simulink model "Controls_Finalproject_1f_linear"  (R2015a)
settings: Solver=ode45  StartTime=0.0  StopTime=1000.0  RelTol=1e-3
values from neighbouring files (symbols this model uses):
  A = [ 0 1 0 0 0 0; 0 0 -(m1*g)/M 0 -m2*g/M 0 ; 0 0 0 1 0 0 ; 0 0 -(M+m1)*g/(M*l1) 0 -m2*g/(M*l1) 0 ; 0 0 0 0 0 1; 0 0 -m1*g/(M*l2) 0 -(M+m2)*g/(M*l2) 0]    [linear_1f.m]    (also in nonlinear_1g.m = [ 0 1 0 0 0 0; 0 0 -(m1*g)/M 0 -m2*g/M 0; 0 0 0 1 0 0; 0 0 -)
  AKL = AKL1    [linear_1f.m]    (also in nonlinear_1g.m)
  B = [0; 1/M; 0; 1/(M*l1); 0; 1/(M*l2)]    [linear_1f.m]    (also in nonlinear_1g.m)
  BL = BL1    [linear_1f.m]    (also in nonlinear_1g.m)
  C = C1    [linear_1f.m]    (also in nonlinear_1g.m)
  CO = eye(6)    [linear_1f.m]    (also in nonlinear_1g.m)
  D = D1    [linear_1f.m]    (also in nonlinear_1g.m)
  DO = DO1    [linear_1f.m]    (also in nonlinear_1g.m)
  X0 = X01    [linear_1f.m]
undefined symbols (not defined in the file or in its folder): K
settings Model: Creator=Aditya Earanky  LastModifiedBy=Vishakha

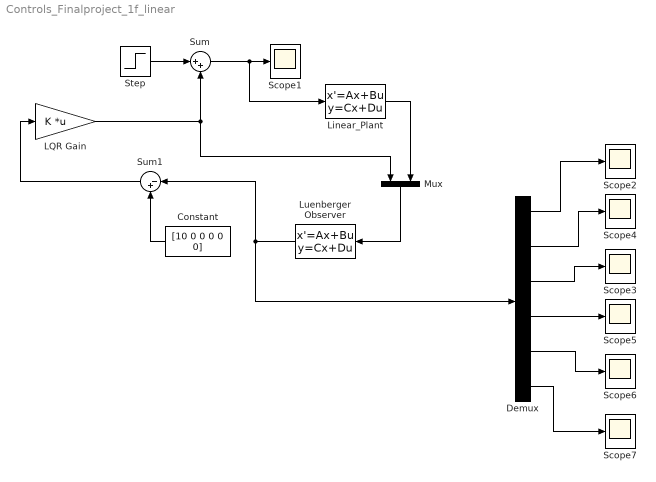
== system Controls_Finalproject_1f_linear ==
  Constant : Constant  Value=[10 0 0 0 0 0]
  Demux : Demux  Outputs=6
  LQR Gain : Gain  Gain=K  Multiplication=Matrix(K*u)
  Linear_Plant : StateSpace  A=A  B=B  C=C  D=D  X0=X0
  Luenberger Observer : StateSpace  A=AKL  B=BL  C=CO  D=DO  X0=0
  Mux : Mux  Inputs=2
  Scope{1..7} (7 alike) : Scope
      Scope1 settings: TimeRange=1000  YMin=0  YMax=0.07
      Scope2 settings: TimeRange=1000  YMin=0  YMax=0.07  SaveName=ScopeData2
      Scope3 settings: TimeRange=1000  YMin=0  YMax=0.07  SaveName=ScopeData3
      Scope4 settings: TimeRange=1000  YMin=0  YMax=0.07  SaveName=ScopeData4
      Scope5 settings: TimeRange=1000  YMin=0  YMax=0.07  SaveName=ScopeData5
      Scope6 settings: TimeRange=1000  YMin=0  YMax=0.07  SaveName=ScopeData6
      Scope7 settings: TimeRange=1000  YMin=0  YMax=0.07  SaveName=ScopeData7
  Step : Step  SampleTime=0
  Sum : Sum  Inputs=|++
  Sum1 : Sum  Inputs=|-+
  wires:
  Linear_Plant/1 -> Mux/2
  Mux/1 -> Luenberger Observer/1
  Luenberger Observer/1 -> Demux/1, Sum1/1
  Sum1/1 -> LQR Gain/1
  Demux/1 -> Scope2/1
  Constant/1 -> Sum1/2
  Demux/2 -> Scope4/1
  Demux/3 -> Scope3/1
  Demux/4 -> Scope5/1
  Demux/5 -> Scope6/1
  Demux/6 -> Scope7/1
  Step/1 -> Sum/1
  LQR Gain/1 -> Sum/2, Mux/1
  Sum/1 -> Linear_Plant/1, Scope1/1
